simulink model "SINGLE_PHASE_BIPOLAR_PWM"  (R2023b)
settings: Solver=VariableStepAuto  StartTime=0.0  StopTime=10.0  RelTol=1e-3
libraries: spsIGBTLib x4, spsDCVoltageSourceLib x1, spsMultimeterLib x1, spsSeriesRLCBranchLib x1, spsTriangleGeneratorLib x1, sps_lib x1
settings Model: Creator=HP5CD  LastModifiedBy=HP5CD

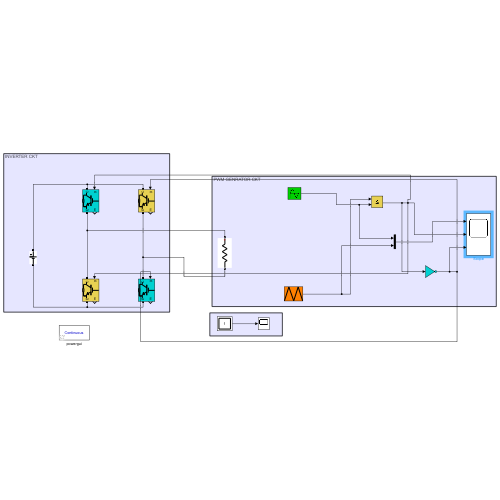
[thumbnail: Simulink's stored preview of the top-level diagram]
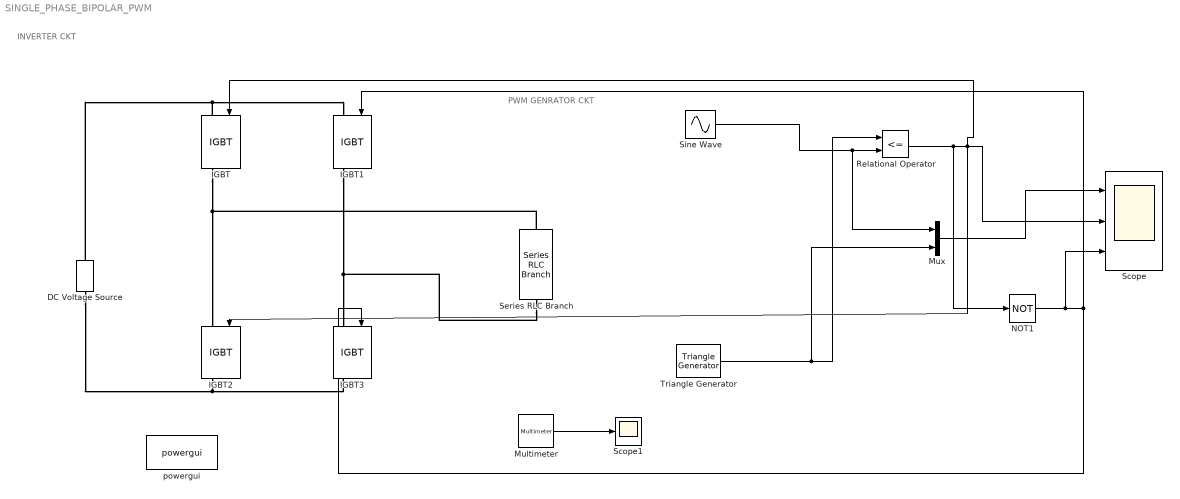
== system SINGLE_PHASE_BIPOLAR_PWM ==
  note: PWM GENRATOR CKT
  note: INVERTER CKT
  DC Voltage Source : spsDCVoltageSourceLib/DC Voltage Source  Amplitude=100  Measurements=None
  IGBT{,1..3} (4 alike) : spsIGBTLib/IGBT  Ron=0.001  Lon=0  Vf=1  Tf=1e-6  Tt=2e-6  IC=0  Rs=1e5  Cs=inf  Measurements=on
  Multimeter : spsMultimeterLib/Multimeter  L=1  sel=1  yselected={}  Gain=1  OutputType=Complex  PlotAtSimulationStop=off  PhasorSimulation=off
  Mux : Mux  Inputs=2
  NOT1 : Logic  Operator=NOT  IconShape=distinctive  AllPortsSameDT=off  OutDataTypeStr=boolean
  Relational Operator : RelationalOperator  Operator=<=  OutDataTypeStr=boolean  RndMeth=Simplest  InputSameDT=off
  Scope : Scope  NumInputPorts=3
  Scope1 : Scope
  Series RLC Branch : spsSeriesRLCBranchLib/Series RLC Branch  LConnTagsString=__new0  RConnTagsString=__new0  BranchType=R  Resistance=1  Inductance=1e-3  SetiL0=off  InitialCurrent=0  Capacitance=1e-6  Setx0=off  InitialVoltage=0  Measurements=Branch voltage
  Sine Wave : Sin  Amplitude=0.8  Frequency=2*pi*50  SampleTime=0
  Triangle Generator : spsTriangleGeneratorLib/Triangle Generator  Freq=1e3  Phase=0  Ts=0
  powergui : sps_lib/powergui  Priority=1  SimulationMode=Continuous  SampleTime=50e-6  frequency=60  Iterations=50  frequencyindice=0  Pbase=100e6  ErrMax=1e-4  UnitsV=kV  UnitsW=MW  buscounter=0  FunctionMessages=off  echomessages=off  EnableUseOfTLC=off  CurrentSourceSwitches=off  DisableSnubberDevices=off  DisableRonSwitches=off  DisableVfSwitches=off  DisplayEquations=off  AutomaticDiscreteSolvers=off  SolverType=Tustin/Backward Euler (TBE)  Interpol=off  ExternalGateDelay=off  methode=off  Ts=100  x0status=blocks  SPID=on  SwTol=0  HookPort=off  NonlinearTolerance=1e-4  nMaxIteration=100  ContinueOnMaxIteration=off  RestoreLinks=warning  ResistiveCurrentMeasurement=off  Frange=[0:2:500]  Ylog=off  Xlog=on  ShowGrid=off  save=off  variable=ZData  structure=0  ZoomFFT=off  StartTime=0.0  cycles=1  DisplayStyle=1  fundamental=60  FreqAxis=off  MaxFrequency=1000  frequencyindicesteady=1  RmsSteady=1  display=off
  wires:
  Sine Wave/1 -> Mux/1, Relational Operator/2
  Triangle Generator/1 -> Mux/2, Relational Operator/1
  Mux/1 -> Scope/1
  Relational Operator/1 -> Scope/2, IGBT/1, IGBT2/1, NOT1/1
  Multimeter/1 -> Scope1/1
  NOT1/1 -> Scope/3, IGBT1/1, IGBT3/1
  connections:
  IGBT/RConn1 -- Series RLC Branch/LConn1 -- IGBT2/LConn1
  IGBT1/RConn1 -- Series RLC Branch/RConn1 -- IGBT3/LConn1
  DC Voltage Source/RConn1 -- IGBT/LConn1 -- IGBT1/LConn1
  DC Voltage Source/LConn1 -- IGBT2/RConn1 -- IGBT3/RConn1
